simulink model "Kd_matrix"  (R2022a)
settings: Solver=VariableStepAuto  StartTime=0.0  StopTime=10.0  RelTol=1e-3
values from neighbouring files (symbols this model uses):
  kd_1 = 500.0    (= 500)    [parameters.m]
  kd_2 = 500.0    (= 500)    [parameters.m]
libraries: matrix_library x2
settings Model: Creator=eleves  LastModifiedBy=eleves

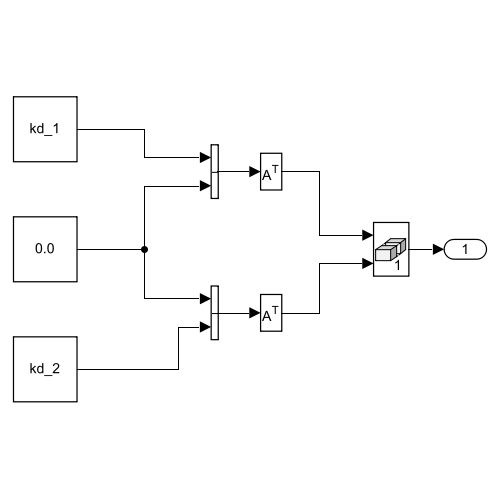
[thumbnail: Simulink's stored preview of the top-level diagram]
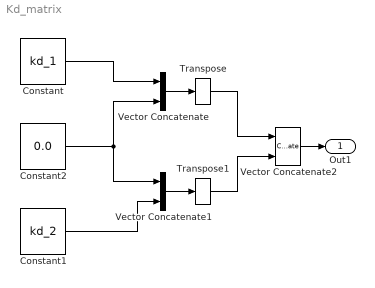
== system Kd_matrix ==
  Constant : Constant  Value=kd_1
  Constant1 : Constant  Value=kd_2
  Constant2 : Constant  Value=0.0
  Transpose : matrix_library/Transpose
      settings: SourceProductBaseCode=SL
  Transpose1 : matrix_library/Transpose
      settings: SourceProductBaseCode=SL
  Vector Concatenate : Concatenate
  Vector Concatenate1 : Concatenate
  Vector Concatenate2 : Concatenate  Mode=Multidimensional array
  Out1 : Outport
  wires:
  Transpose1/1 -> Vector Concatenate2/2
  Transpose/1 -> Vector Concatenate2/1
  Constant/1 -> Vector Concatenate/1
  Constant1/1 -> Vector Concatenate1/2
  Vector Concatenate/1 -> Transpose/1
  Vector Concatenate1/1 -> Transpose1/1
  Vector Concatenate2/1 -> Out1/1
  Constant2/1 -> Vector Concatenate/2, Vector Concatenate1/1
